simulink model "hydrooo"  (R2013a)
settings: Solver=ode45  StartTime=0.0  StopTime=100  RelTol=1e-3
settings Model: Creator=SAITFASKA  LastModifiedBy=SAITFASKA

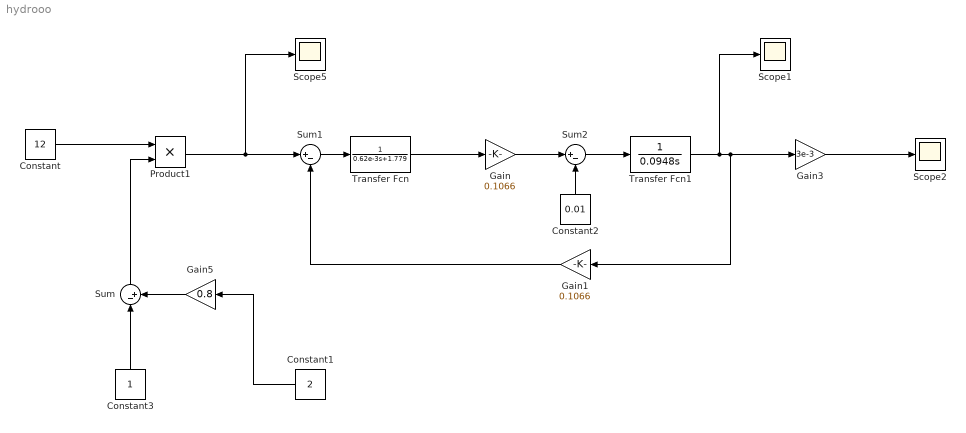
== system hydrooo ==
  Constant : Constant  Value=12
  Constant1 : Constant  Value=2
  Constant2 : Constant  Value=0.01
  Constant3 : Constant
  Gain : Gain  Gain=0.1066
  Gain1 : Gain  Gain=0.1066
  Gain3 : Gain  Gain=3e-3
  Gain5 : Gain  Gain=0.8
  Product1 : Product
  Scope1 : Scope
      settings: YMin=411.666  YMax=455
  Scope2 : Scope
      settings: SaveName=ScopeData2
  Scope5 : Scope
      settings: YMin=54  YMax=58.5  SaveName=ScopeData5
  Sum : Sum  Inputs=|-+
  Sum1 : Sum  Inputs=|+-
  Sum2 : Sum  Inputs=|+-
  Transfer Fcn : TransferFcn  Denominator="[0.62e-3  1.779]"
  Transfer Fcn1 : TransferFcn  Denominator=[ 0.0948 0]
  wires:
  Gain/1 -> Sum2/1
  Sum2/1 -> Transfer Fcn1/1
  Sum1/1 -> Transfer Fcn/1
  Gain1/1 -> Sum1/2
  Transfer Fcn1/1 -> Scope1/1, Gain3/1, Gain1/1
  Constant2/1 -> Sum2/2
  Transfer Fcn/1 -> Gain/1
  Constant/1 -> Product1/1
  Product1/1 -> Sum1/1, Scope5/1
  Sum/1 -> Product1/2
  Gain5/1 -> Sum/2
  Gain3/1 -> Scope2/1
  Constant1/1 -> Gain5/1
  Constant3/1 -> Sum/1
